simulink model "VTOL"  (R2016b)
settings: Solver=VariableStepAuto  StartTime=0.0  StopTime=50.0  RelTol=1e-3  EnableMultiTasking=on
libraries: vrlib x3, simulink_extras x1, simulink x1
settings Model: Creator=AI  LastModifiedBy=Matthias
settings OptimizationCC: LifeSpan=inf
settings DebuggingCC: SFUnexpectedBacktrackingDiag=warning  SFNoUnconditionalDefaultTransitionDiag=warning  SFExecutionAtInitializationDiag=none
settings GRTTargetCC: TargetLangStandard=C89/C90 (ANSI)  GeneratePreprocessorConditionals=Disable all
settings ConfigComp: CovMetricSettings=dw  CovHtmlReporting=on  CovSaveCumulativeToWorkspaceVar=on  CovSaveSingleToWorkspaceVar=on  CovExternalEMLEnable=off

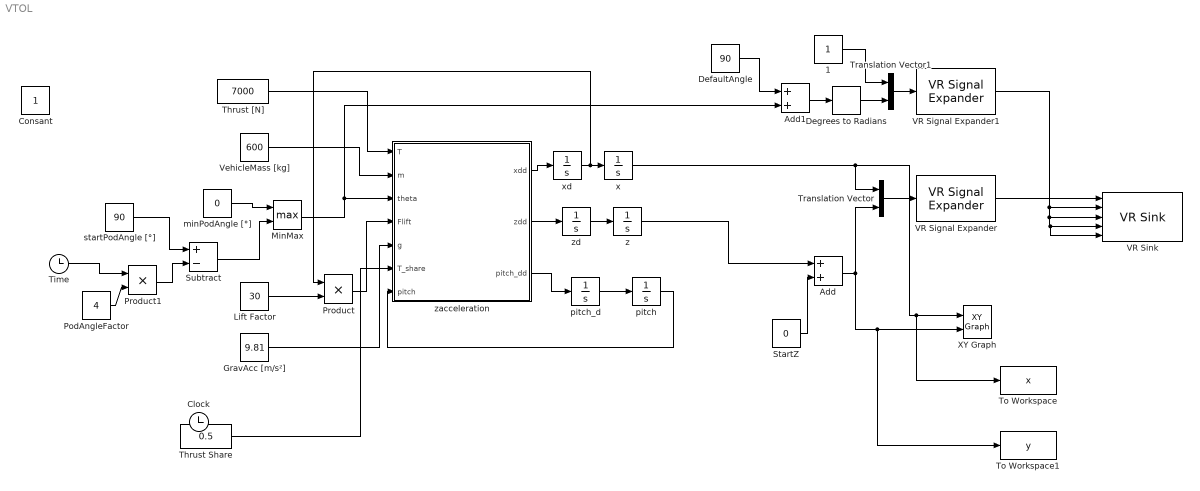
== system VTOL ==
  1 : Constant
  Add : Sum
  Add1 : Sum
  DefaultAngle : Constant  Value=90
  Degrees to Radians : simulink_extras/Transformations/Degrees to Radians
  GravAcc [m/s²] : Constant  Value=9.81
  Lift Factor : Constant  Value=30
  MinMax : MinMax  Function=max  Inputs=2
  PodAngleFactor : Constant  Value=4
  Product : Product
  Product1 : Product
  StartZ : Constant  Value=0
  Subtract : Sum  Inputs=+-
  Thrust Share : Constant  Value=0.5
  Thrust [N] : Constant  Value=7000
  Time : Clock
  To Workspace : ToWorkspace  VariableName=x  SampleTime=-1
  To Workspace1 : ToWorkspace  VariableName=y  SampleTime=-1
  Translation Vector : Concatenate
  Translation Vector1 : Concatenate
  VR Signal Expander : vrlib/VR Signal Expander  outwidth=3  outidx=[1 2]
  VR Signal Expander1 : vrlib/VR Signal Expander  outwidth=4  outidx=[3 4]
  VR Sink : vrlib/VR Sink  InstantiateOnLoad=on  SampleTime=0.01  ViewEnable=on  RemoteChange=off  RemoteView=off  FieldsWritten=Flutr.translation.3.1.1.double#Pod1.rotation.4.1.1.double#Pod2.rotation.4.1.1.double#Pod3.rotation.4.1.1.double#Pod4.rotation.4.1.1.double  WorldFileName=VRfileFlutr.wrl  AutoView=off  VideoDimensions=[]  AllowVariableSize=off
  VehicleMass [kg] : Constant  Value=600
  XY Graph : simulink/Sinks/XY Graph  xmin=-1  xmax=10000  ymin=-1  ymax=1000  st=-1
  minPodAngle [°] : Constant  Value=0
  pitch : Integrator
  pitch_d : Integrator
  startPodAngle [°] : Constant  Value=90
  x : Integrator
  xd : Integrator
  z : Integrator
  zacceleration : MATLAB Function  TreatAsAtomicUnit=on
  zd : Integrator
  Clock : Clock
      settings: IOType=siggen
  Consant : Constant  IOType=siggen
  wires:
  Thrust [N]/1 -> zacceleration/1(T)
  VehicleMass [kg]/1 -> zacceleration/2(m)
  xd/1 -> Product/1, x/1
  GravAcc [m/s²]/1 -> zacceleration/5(g)
  zd/1 -> z/1
  zacceleration/2(zdd) -> zd/1
  z/1 -> Add/1
  Lift Factor/1 -> Product/2
  Product/1 -> zacceleration/4(Flift)
  Translation Vector/1 -> VR Signal Expander/1
  x/1 -> To Workspace/1, XY Graph/1, Translation Vector/1
  StartZ/1 -> Add/2
  Add/1 -> Translation Vector/2, To Workspace1/1, XY Graph/2
  VR Signal Expander/1 -> VR Sink/1
  VR Signal Expander1/1 -> VR Sink/5, VR Sink/4, VR Sink/3, VR Sink/2
  Translation Vector1/1 -> VR Signal Expander1/1
  1/1 -> Translation Vector1/1
  Degrees to Radians/1 -> Translation Vector1/2
  DefaultAngle/1 -> Add1/1
  Add1/1 -> Degrees to Radians/1
  zacceleration/1(xdd) -> xd/1
  MinMax/1 -> Add1/2, zacceleration/3(theta)
  minPodAngle [°]/1 -> MinMax/1
  startPodAngle [°]/1 -> Subtract/1
  Subtract/1 -> MinMax/2
  Product1/1 -> Subtract/2
  PodAngleFactor/1 -> Product1/2
  Time/1 -> Product1/1
  zacceleration/3(pitch_dd) -> pitch_d/1
  pitch_d/1 -> pitch/1
  pitch/1 -> zacceleration/7(pitch)
  Thrust Share/1 -> zacceleration/6(T_share)

== matlab function VTOL/zacceleration ==
  data: xdd output; T input; zdd output; m input; theta input; Flift input; g input; T_share input; pitch_dd output; pitch input
function [xdd, zdd,pitch_dd] = accel(T,m,theta,Flift,g,T_share,pitch) 
%T_share: percentage of Thrust put to the bottom pods, i.e. T_share = 0.6
%=> 40% rear pod thrust, 60% bottom pod thrust
%#codegen
xdd=cos(theta*pi/180 + pitch)*T/m;
zdd=sin(theta*pi/180 + pitch)*T/m+Flift/m-g;
% h_1, x_1: Distance from forward pods to CG
% h_2, x_2: Distance from rear pods to CG
h_1 = 1;
h_2 = 1;
x_1 = 2;
x_2 = 2;
% I: Moment of inertia
I = 50;
pitch_dd = (cos(theta*pi/180 + pitch) * T * (h_1*(1-T_share) - h_2*T_share) + sin(theta*pi/180 + pitch) * T * (x_1*(1-T_share) - x_2*T_share)) / I;
% Todo pitch_dd
